simulink model "PID_LP"  (R2023b)
settings: Solver=VariableStepAuto  StartTime=0.0  StopTime=10.0  RelTol=1e-3
values from neighbouring files (symbols this model uses):
  beta = 0.65    [pid_lp_parameters.m]    (also in plant.m = 0.05; plant_2.m = 0.7)
  fd = 183    [pid_lp_parameters.m]
  kp = 32000000    [pid_lp_parameters.m]    (also in plant.m = 10; plant_2.m = 10)
  wlp = 2*pi*flp    (= 31415.9265359)    [pid_lp_parameters.m]
undefined symbols (not defined in the file or in its folder): Kp
settings Model: Creator=anandsingh  LastModifiedBy=anandsingh

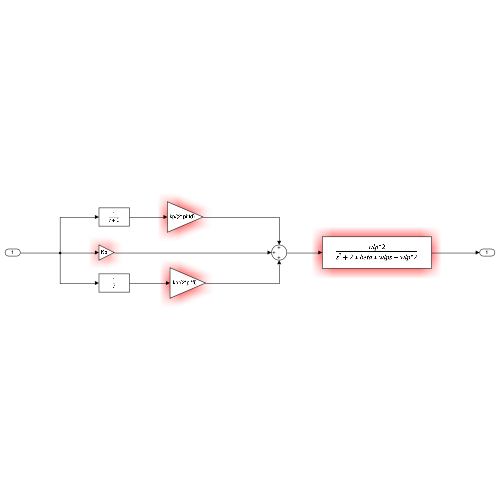
[thumbnail: Simulink's stored preview of the top-level diagram]
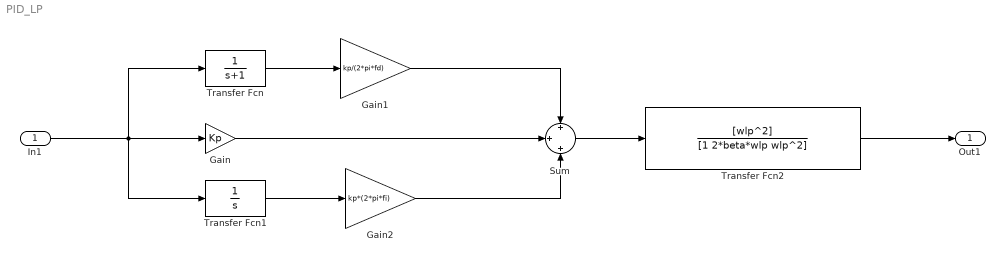
== system PID_LP ==
  In1 : Inport
  Gain : Gain  Gain=Kp
  Gain1 : Gain  Gain=kp/(2*pi*fd)
  Gain2 : Gain  Gain=kp*(2*pi*fi)
  Sum : Sum  Inputs=+|+|+
  Transfer Fcn : TransferFcn  Denominator=[1 1]
  Transfer Fcn1 : TransferFcn  Denominator=[1 0]
  Transfer Fcn2 : TransferFcn  Numerator=[wlp^2]  Denominator=[1 2*beta*wlp wlp^2]
  Out1 : Outport
  wires:
  Gain1/1 -> Sum/1
  Gain/1 -> Sum/2
  Gain2/1 -> Sum/3
  Sum/1 -> Transfer Fcn2/1
  Transfer Fcn/1 -> Gain1/1
  Transfer Fcn1/1 -> Gain2/1
  In1/1 -> Transfer Fcn/1, Transfer Fcn1/1, Gain/1
  Transfer Fcn2/1 -> Out1/1
